simulink model "GaitAlgorithm_arduino_V1"  (R2024a)
settings: Solver=FixedStepAuto  StartTime=0.0  StopTime=inf  RelTol=1e-3  EnableMultiTasking=on
undefined symbols (not defined in the file): DiscIntNeverNeededParam
libraries: simulink x26, mcp2515lib x13, matrix_library x6, arduinolib x2, arduinosensorlib x2
(part 1 of 2)
settings Model: ExtModeTrigDuration=2  Creator=82108  LastModifiedBy=sejon
settings OptimizationCC: EnhancedBackFolding=on  PassReuseOutputArgsAs=Individual arguments  ZeroExternalMemoryAtStartup=off  ZeroInternalMemoryAtStartup=off  MaxStackSize=64  OptimizeBlockOrder=speed  DifferentSizesBufferReuse=on  OptimizationCustomize=off  EfficientTunableParamExpr=on
settings DebuggingCC: ParameterTunabilityLossMsg=error
settings HardwareCC: ProdBitPerInt=16  ProdBitPerPointer=16  ProdBitPerSizeT=16  ProdBitPerPtrDiffT=16  ProdLargestAtomicFloat=None  ProdWordSize=8  ProdHWDeviceType=Atmel->AVR  TargetBitPerPointer=64  TargetBitPerSizeT=64  TargetBitPerPtrDiffT=64  TargetLongLongMode=on  TargetIntDivRoundTo=Zero  TargetEndianess=LittleEndian  TargetWordSize=64  TargetHWDeviceType=Custom Processor->MATLAB Host Computer  ProdEqTarget=off
settings SFSimCC: MATLABDynamicMemAlloc=off
settings RTWCC: Description=Embedded Coder  SystemTargetFile=ert.tlc  HardwareBoard=Arduino Uno  TemplateMakefile=ert_default_tmf  Toolchain=Arduino AVR  BuildConfiguration=Faster Runs  GPUComputeCapability=3.5
settings CodeAppCC: ForceParamTrailComments=on  IgnoreCustomStorageClasses=off  OperatorAnnotations=on  SimulinkDataObjDesc=on  SFDataObjDesc=on  InsertBlockDesc=on
settings ERTTargetCC: SupportContinuousTime=on  SupportVariableSizeSignals=on  ExtModeTransport=3  ExtModeStaticAlloc=on  ExtModeAutomaticAllocSize=off  ExtModeStaticAllocSize=250  ExtModeMexFile=ext_xcp  ExtModeIntrfLevel=Level2 - Open

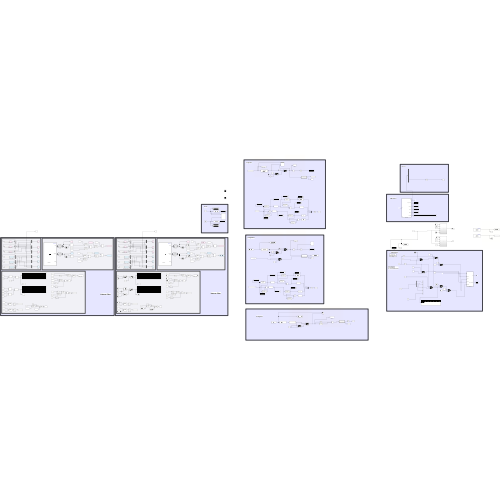
[thumbnail: Simulink's stored preview of the top-level diagram]
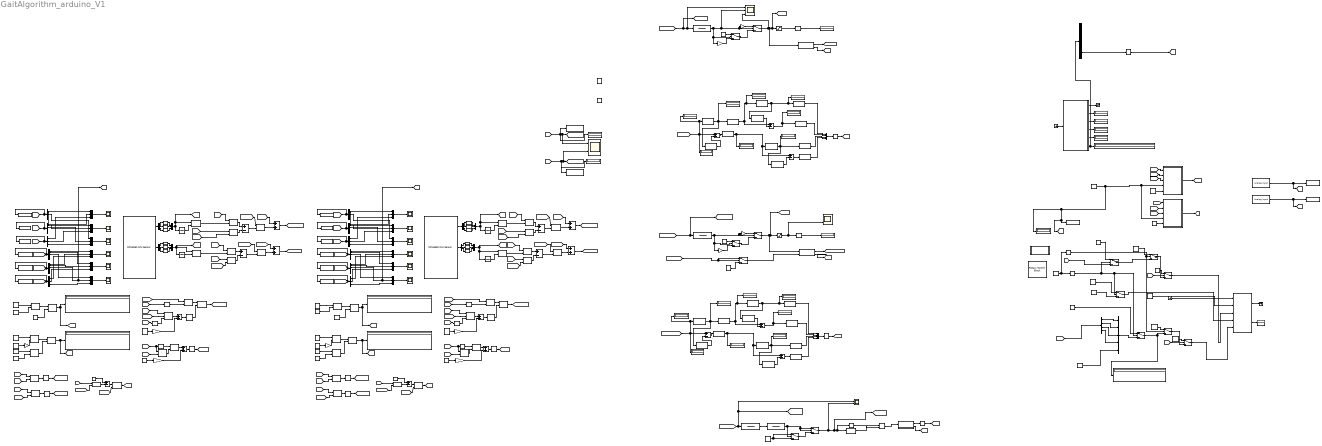
== system GaitAlgorithm_arduino_V1 ==
  note: D : Driving Mode
      | Z : Zeroing Mode
      | TZ : To zero Position Mode
  note: LIMIT STOP
  note: CAN Transmit
  note: DC Algorithm
  note: IC Algorithm
  note: Kalman Filter
  note: IMU data
  note: CAN Receive
  note: IC
  note: Kalman Filter
  note: LG Algorithm
  AND2 : Logic  IconShape=distinctive  AllPortsSameDT=off  OutDataTypeStr=boolean
  Acc_x : Scope
  Acc_x1 : Scope
  Acc_y : Scope
  Acc_y1 : Scope
  Acc_z : Scope
  Acc_z1 : Scope
  Add{,1,6,9..10,13..15} (8 alike) : Sum
  Add{2..5,7..8,11..12,16..19} (12 alike) : Sum  Inputs=+-
  Analog Input : arduinolib/Analog Input  pinNumber=0  ReadResultsOnly=off  ConversionTriggerSource=Software  ExternalTriggerType=uint32( 0 )  OutputDataType=uint16  EnableConversionCompleteNotify=off  EnableOuputStatus=off  SampleTime=0.01  blockPlatform=arduino
  Analog Input1 : arduinolib/Analog Input  pinNumber=1  ReadResultsOnly=off  ConversionTriggerSource=Software  ExternalTriggerType=uint32( 0 )  OutputDataType=uint16  EnableConversionCompleteNotify=off  EnableOuputStatus=off  SampleTime=0.01  blockPlatform=arduino
  Bias{,1..11} (12 alike) : Bias  SaturateOnIntegerOverflow=off
  CANbegin : Subsystem  TreatAsAtomicUnit=on  mask{TargetHardware=Arduino, Oscillator=8, CANSpeed=1000, CSpin=10}
      mask prompts: TargetHardware "Target Hardware"; Oscillator "Oscillator frequency(MHz)"; CANSpeed "CAN speed(kHz)"; CSpin "Chip Select Pin"
      mask init:
      | % Get this mask's handle
      | maskObj = Simulink.Mask.get(gcb);
      | 
      | % Get the selected value from mask parameter's option
      | str_TargetHard = char(maskObj.Parameters(1).TypeOptions(TargetHardware));
      | str_Osc = char(maskObj.Parameters(2).TypeOptions(Oscillator));
      | str_CANSpeed = char(maskObj.Parameters(3).TypeOptions(CANSpeed));
      | 
      | % Set Icon
      | str1 = sprintf('%s(Model)',str_TargetHard);
      | str2 = sprintf('Oscillator: %s(MHz)',str_Osc);
      | str3 = sprintf('CAN Bus Speed: %s(kHz)',str_CANSpeed);
      | str4 = sprintf('Chip Select pin: %d',CSpin);
      | 
      | % Set the values of Variant Subsystem
      | switch str_TargetHard
      |     case 'Arduino'
      |         str = [str1,'\n',str2,'\n',str3,'\n',str4];
      |         evalin('base',sprintf('CSpin = %d;',CSpin));        
      |         evalin('base','Hardware = 1;');
      |     case 'Raspberry Pi'
      |         str = [str1,'\n',str2,'\n',str3];
      |         evalin('base',sprintf('clear CSpin',CSpin));           
      |         evalin('base','Hardware = 2;');     
      | end  
      | 
      | % Get the CAN Configuration register's value from mask parameter's option
      | if str_Osc == '8' %[MHz]
      |     switch str_CANSpeed
      |         case '1000'
      |             BPR = 0; PHSEG1 = 0; PRSEG = 0; PHSEG2 = 0;
      |         case '500'
      |             BPR = 0; PHSEG1 = 2; PRSEG = 0; PHSEG2 = 2;
      |         case '250'
      |             BPR = 0; PHSEG1 = 6; PRSEG = 0; PHSEG2 = 6;
      |         case '125'
      |             BPR = 1; PHSEG1 = 6; PRSEG = 1; PHSEG2 = 5;
      |         case '100'
      |             BPR = 1; PHSEG1 = 7; PRSEG = 2; PHSEG2 = 7;
      |         case '83.3'
      |             BPR = 1; PHSEG1 = 7; PRSEG = 6; PHSEG2 = 7;
      |         case '62.5'
      |             BPR = 3; PHSEG1 = 6; PRSEG = 0; PHSEG2 = 6;
      |         case '50'
      |             BPR = 3; PHSEG1 = 7; PRSEG = 2; PHSEG2 = 7;
      |         case '33.3'
      |             BPR = 4; PHSEG1 = 7; PRSEG = 6; PHSEG2 = 7;
      |     end            
      | elseif str_Osc == '16' %[MHz]
      |     switch str_CANSpeed  
      |         case '1000'
      |             BPR = 0; PHSEG1 = 2; PRSEG = 0; PHSEG2 = 2;
      |         case '500'
      |             BPR = 0; PHSEG1 = 6; PRSEG = 0; PHSEG2 = 6;
      |         case '250'
      |             BPR = 1; PHSEG1 = 6; PRSEG = 1; PHSEG2 = 5;        
      |         case '125'
      |             BPR = 3; PHSEG1 = 6; PRSEG = 0; PHSEG2 = 6;
      |         case '100'
      |             BPR = 3; PHSEG1 = 7; PRSEG = 2; PHSEG2 = 7;
      |         case '83.3'
      |             BPR = 3; PHSEG1 = 7; PRSEG = 6; PHSEG2 = 7;
      |         case '62.5'
      |             BPR = 7; PHSEG1 = 6; PRSEG = 0; PHSEG2 = 6;
      |         case '50'
      |             BPR = 7; PHSEG1 = 7; PRSEG = 2; PHSEG2 = 7;
      |         case '33.3'
      |             BPR = 9; PHSEG1 = 7; PRSEG = 6; PHSEG2 = 7;        
      |     end   
      | end
      | % Set the CAN Configuration register's value
      | address2A = BPR;          % bit7-6 :SJW, bit5-0: BPR
      | address29 = 192 ...       % bit7: BTLMODE = 1, bit6:SAM = 1
      |             + 8*PHSEG1 ...% bit5-3: PHSEG1
      |             +PRSEG;       % bit2-0: PRSEG
      | address28 = 128 ...       % bit7: SOF = 1, bit6:WAKFIL = 0
      |             + PHSEG2;     % bit5-3: 0, bit2-0: PHSEG2
      settings: RTWSystemCode=Nonreusable function
      mask TypeOptions TargetHardware: Arduino | Raspberry Pi
      mask Callback TargetHardware:
      | if(strcmp(get_param(gcb,'TargetHardware'),'Arduino'))
      |     set_param(gcb,'MaskVisibilities',{'on','on','on','on'})
      | else
      |     set_param(gcb,'MaskVisibilities',{'on','on','on','off'})
      | end
      mask TypeOptions Oscillator: 8 | 16
      mask TypeOptions CANSpeed: 1000 | 500 | 250 | 125 | 100 | 83.3 | 62.5 | 50 | 33.3
      mask DialogControl DescGroupVar Prompt: Description
      mask DialogControl DescTextVar Prompt: This block must be executed only once when beginning CAN communication because MCP2515’s register needs to be configured. And the frequency of oscillator for MCP2515 is also needed because it effects to the setting parameters of MCP2515's register.
      mask Display: disp(str)
  CANreceive : Subsystem  TreatAsAtomicUnit=on
      mask DialogControl DescGroupVar Prompt: Description
      mask DialogControl DescTextVar Prompt: CANreceive outputs CAN data by converting MCP2515 RX buffer register’s values. In/Out ports are no use because they are used for controlling the execution order. CAN_Received outputs 1(CAN received) or -1( No message).
  CANtransmit : Subsystem  TreatAsAtomicUnit=on
      mask DialogControl DescGroupVar Prompt: Description
      mask DialogControl DescTextVar Prompt: CANtransmit inputs CAN data by converting MCP2515 TX buffer register’s values. In/Out ports are no use because they are used for controlling the execution order. CAN_Transmitted outputs 1(Success) or 2(Fail).
  Compare To Constant1 : simulink/Logic and Bit Operations/Compare To Constant  relop=>=  const=0  OutDataTypeStr=boolean
  Compare To Constant4 : simulink/Logic and Bit Operations/Compare To Constant  relop=>=  const=0  OutDataTypeStr=boolean
  Compare To Constant5 : simulink/Logic and Bit Operations/Compare To Constant  relop=>  const=-2  OutDataTypeStr=boolean
  Compare To Constant7 : simulink/Logic and Bit Operations/Compare To Constant  relop===  const=1  OutDataTypeStr=boolean
  Compare To Constant8 : simulink/Logic and Bit Operations/Compare To Constant  relop===  const=2  OutDataTypeStr=boolean
  Compare To Constant9 : simulink/Logic and Bit Operations/Compare To Constant  relop=>=  const=0xff  OutDataTypeStr=boolean
  Constant : Constant  Value=[0 0 0 0]  OutDataTypeStr=uint8
  Constant1 : Constant  OutDataTypeStr=uint8
  Constant10 : Constant  Value=[0 0 0; 0 0 0; 0 0 0]  SampleTime=-1
  Constant11 : Constant  Value=[0 0 0; 0 0 0; 0 0 0]
  Constant12 : Constant  Value=[0 0 0 0 0 0; 0 0 0 0 0 0; 0 0 0 0 0 0]
  Constant13 : Constant  Value=[0 0 0; 0 0 0; 0 0 0]
  Constant14 : Constant  Value=0x168  OutDataTypeStr=uint16
  Constant15 : Constant  Value=[0x00 0x00 0x07 0xd0 ]  OutDataTypeStr=uint16
  Constant16 : Constant  Value=-1
  Constant17 : Constant  Value=-1
  Constant18 : Constant  Value=-2
  Constant19 : Constant  Value=3  SampleTime=0.01
  Constant21 : Constant  Value=0x468
  Constant22 : Constant  Value=[0 0 0 0 0 0 0 0 ]  OutDataTypeStr=uint8
  Constant23 : Constant  Value=0x468
  Constant24 : Constant  Value=[0 0 0 0 0 0 0 0 ]  OutDataTypeStr=uint8
  Constant25 : Constant  Value=2
  Constant3 : Constant  Value=4  OutDataTypeStr=uint8
  Constant4 : Constant  Value=-10
  Constant5 : Constant  Value=0x568
  Constant6 : Constant  OutDataTypeStr=uint8
  Constant7 : Constant  Value=[0x01 0 0 0 0 0 0 0]  OutDataTypeStr=uint8
  Constant8 : Constant  Value=[0 0 0; 0 0 0; 0 0 0]
  Constant9 : Constant  Value=[0 0 0 0 0 0; 0 0 0 0 0 0; 0 0 0 0 0 0]  SampleTime=-1
  Data Store Memory : DataStoreMemory  DataStoreName=T_G_Z  WriteAfterWriteMsg=warning  ShowAdditionalParam=off
  Data Store Memory1 : DataStoreMemory  DataStoreName=S_G_Z  WriteAfterWriteMsg=warning  ShowAdditionalParam=off
  Data Store Write : DataStoreWrite  DataStoreName=T_G_Z  DataStoreElements=T_G_Z  IndexOptions=Index vector (dialog)  Indices=1  OutputSizes=1
  Data Store Write1 : DataStoreWrite  DataStoreName=S_G_Z  DataStoreElements=S_G_Z  IndexOptions=Index vector (dialog)  Indices=1  OutputSizes=1
  Data Type Conversion{1..2,10..11} (4 alike) : DataTypeConversion  OutDataTypeStr=uint16  SaturateOnIntegerOverflow=off  RndMeth=Floor
  Data Type Conversion{6..7,9,12} (4 alike) : DataTypeConversion  OutDataTypeStr=uint8  SaturateOnIntegerOverflow=off  RndMeth=Floor
  Data Type Conversion{3..5,8} (4 alike) : DataTypeConversion  OutDataTypeStr=uint8  RndMeth=Floor
  Delay1 : Delay  DelayLength=1
  Delay2 : Delay  DelayLength=1
  Delay_acc : Delay  DelayLength=1  InitialCondition=[0; 0; 0; 0; 0;0]
  Delay_acc1 : Delay  DelayLength=1  InitialCondition=[0; 0; 0; 0; 0;0]
  Delay_gyro : Delay  DelayLength=1  InitialCondition=[0; 0; 0; 0; 0;0]
  Delay_gyro1 : Delay  DelayLength=1  InitialCondition=[0; 0; 0; 0; 0;0]
  Demux : Demux  Outputs=8
  Demux{3..4,6..7,9..10,16,18} (8 alike) : Demux  Outputs=6
  Demux{5,8,11..15,17} (8 alike) : Demux  Outputs=3
  Demux2 : Demux
  Detect Increase1 : simulink/Logic and Bit Operations/Detect Increase  vinit=0.0  OutDataTypeStr=boolean
  Discrete-Time Integrator{,1..3} (4 alike) : DiscreteIntegrator  SampleTime=-1  ICPrevOutput=DiscIntNeverNeededParam  ICPrevScaledInput=DiscIntNeverNeededParam
  Display{1..24,27..33} (31 alike) : Display
      Display11 settings: Format=hex (Stored Integer)
      Display12 settings: Format=hex (Stored Integer)
      Display13 settings: Format=hex (Stored Integer)
      Display14 settings: Format=hex (Stored Integer)
      Display15 settings: Format=hex (Stored Integer)
      Display16 settings: Format=hex (Stored Integer)
      Display17 settings: Format=hex (Stored Integer)
      Display18 settings: Format=hex (Stored Integer)
      Display19 settings: Format=hex (Stored Integer)
      Display20 settings: Format=hex (Stored Integer)
      Display21 settings: Format=hex (Stored Integer)
      Display22 settings: Format=hex (Stored Integer)
      Display23 settings: Format=hex (Stored Integer)
      Display24 settings: Format=hex (Stored Integer)
      Display28 settings: Format=hex (Stored Integer)
      Display30 settings: Format=hex (Stored Integer)
      Display32 settings: Format=hex (Stored Integer)
      Display7 settings: Format=hex (Stored Integer)
      Display9 settings: Format=hex (Stored Integer)
  Enabled Subsystem1 : Subsystem  TreatAsAtomicUnit=on
  Enabled Subsystem3 : Subsystem  TreatAsAtomicUnit=on
  Enabled Subsystem4 : Subsystem  TreatAsAtomicUnit=on
  Gain : Gain  Gain=-0.01
  Gain1 : Gain  Gain=-0.01
  Gain{2..5} (4 alike) : Gain  Gain=2
  Ground : Ground
  Ground1 : Ground
  Gyro_x : Scope
  Gyro_x1 : Scope
  Gyro_y : Scope
  Gyro_y1 : Scope
  Gyro_z : Scope
  Gyro_z1 : Scope
  IdentityMatrix{,1..2,4,7..9,11} (8 alike) : IdentityMatrix  OutputDimensions=3  SampleTime=-1
  IdentityMatrix{3,5..6,10,12..13} (6 alike) : IdentityMatrix  OutputDimensions=6  SampleTime=-1
  MPU6050 IMU Sensor : arduinosensorlib/MPU6050 IMU Sensor  I2CModule=0  SlaveAddress=0x68  Accel=on  AngularRate=on  Temperature=off  Status=on  Timestamp=off  EulerAngles=off  Quat=off  AccelRange=2G  GyroRange=250 dps  DmpOdr=200 Hz  Dlpf=Accelerometer: 184Hz, Gyroscope: 188Hz  spf=1  SampleTime=0.01  QueueSizeFactor=1
  MPU6050 IMU Sensor1 : arduinosensorlib/MPU6050 IMU Sensor  I2CModule=0  SlaveAddress=0x69  Accel=on  AngularRate=on  Temperature=off  Status=on  Timestamp=off  EulerAngles=off  Quat=off  AccelRange=2G  GyroRange=250 dps  DmpOdr=200 Hz  Dlpf=Accelerometer: 184Hz, Gyroscope: 188Hz  spf=1  SampleTime=0.01  QueueSizeFactor=1
  Matrix Concatenate{,1,4,7..8,11} (6 alike) : Concatenate  Mode=Multidimensional array  ConcatenateDimension=2
  Matrix Concatenate{2..3,5..6,9..10,12..13} (8 alike) : Concatenate  Mode=Multidimensional array
  Matrix Divide : Product  Inputs=/  Multiplication=Matrix(*)
  Matrix Divide1 : Product  Inputs=/  Multiplication=Matrix(*)
  Matrix Multiply{,1..3,5..23,25..29} (28 alike) : Product  Multiplication=Matrix(*)
  Matrix Multiply24 : Product  Inputs=3  Multiplication=Matrix(*)
  Matrix Multiply4 : Product  Inputs=3  Multiplication=Matrix(*)
  Mux{,1..15} (16 alike) : Mux  Inputs=3
  Reshape1 : Reshape
  Reshape2 : Reshape
  Reshape3 : Reshape
  Rotary Switch : RotarySwitchBlock
      settings: Values={{'D', 'Z', 'TZ'}, [0 1 2]}
  Saturation1 : Saturate  UpperLimit=200  LowerLimit=-100
  Saturation3 : Saturate  UpperLimit=200  LowerLimit=-100
  Scope : Scope  NumInputPorts=2
  Scope1 : Scope  NumInputPorts=2
  Scope3 : Scope  NumInputPorts=3
  Scope4 : Scope  NumInputPorts=2
  Shift Arithmetic{1,7,10..11} (4 alike) : ArithShift  BitShiftNumber=8  BitShiftDirection=Right
  Shift Arithmetic13 : ArithShift  BitShiftNumber=16  BitShiftDirection=Right
  Shift Arithmetic{2,4,6,9} (4 alike) : ArithShift  BitShiftNumber=8  BitShiftDirection=Left
  Shift Arithmetic3 : ArithShift  BitShiftNumber=16  BitShiftDirection=Left
  Shift Arithmetic5 : ArithShift  BitShiftNumber=16  BitShiftDirection=Right
  Shift Arithmetic8 : ArithShift  BitShiftNumber=16  BitShiftDirection=Left
  Subsystem : Subsystem
  Subsystem1 : Subsystem
  Switch{,1..4,11..12} (7 alike) : Switch  Criteria=u2 > Threshold  SaturateOnIntegerOverflow=off  InputSameDT=off
  Switch10 : Switch  Threshold=2  SaturateOnIntegerOverflow=off  InputSameDT=off
  Switch13 : Switch  Criteria=u2 > Threshold  Threshold=25  SaturateOnIntegerOverflow=off  InputSameDT=off
  Switch5 : Switch  Criteria=u2 > Threshold  Threshold=40  SaturateOnIntegerOverflow=off  InputSameDT=off
  Switch6 : Switch  Criteria=u2 > Threshold  Threshold=-40  SaturateOnIntegerOverflow=off  InputSameDT=off
  Switch7 : Switch  Criteria=u2 > Threshold  Threshold=10  SaturateOnIntegerOverflow=off  InputSameDT=off
  Switch8 : Switch  Criteria=u2 > Threshold  Threshold=-10  SaturateOnIntegerOverflow=off  InputSameDT=off
  Switch9 : Switch  Threshold=-2  SaturateOnIntegerOverflow=off  InputSameDT=off
  Terminator : Terminator
  Terminator1 : Terminator
  To Workspace : ToWorkspace  VariableName=predicted_acc  SaveFormat=Timeseries  SampleTime=-1
  To Workspace1 : ToWorkspace  VariableName=measured_acc  SaveFormat=Timeseries  SampleTime=-1
  To Workspace10 : ToWorkspace  VariableName=estimated_gyro_shank  SaveFormat=Timeseries  SampleTime=-1
  To Workspace11 : ToWorkspace  VariableName=measured_gyro_shank  SaveFormat=Timeseries  SampleTime=-1
  To Workspace12 : ToWorkspace  VariableName=UDPsig  SaveFormat=Timeseries  SampleTime=-1
  To Workspace13 : ToWorkspace  VariableName=emg0  SaveFormat=Timeseries  SampleTime=-1
  To Workspace14 : ToWorkspace  VariableName=emg1  SaveFormat=Timeseries  SampleTime=-1
  To Workspace2 : ToWorkspace  VariableName=estimated_acc  SaveFormat=Timeseries  SampleTime=-1
  To Workspace3 : ToWorkspace  VariableName=predicted_gyro  SaveFormat=Timeseries  SampleTime=-1
  To Workspace4 : ToWorkspace  VariableName=estimated_gyro  SaveFormat=Timeseries  SampleTime=-1
  To Workspace5 : ToWorkspace  VariableName=measured_gyro  SaveFormat=Timeseries  SampleTime=-1
  To Workspace6 : ToWorkspace  VariableName=predicted_acc_shank  SaveFormat=Timeseries  SampleTime=-1
  To Workspace7 : ToWorkspace  VariableName=measured_acc_shank  SaveFormat=Timeseries  SampleTime=-1
  To Workspace8 : ToWorkspace  VariableName=estimated_acc_shank  SaveFormat=Timeseries  SampleTime=-1
  To Workspace9 : ToWorkspace  VariableName=predicted_gyro_shank  SaveFormat=Timeseries  SampleTime=-1
  Transfer Fcn1 : TransferFcn  Denominator=[0.029 1]
  Transfer Fcn18 : TransferFcn  Numerator=[0.018 0]  Denominator=[0.018 1]
  Transfer Fcn19 : TransferFcn  Denominator=[0.08 1]
  Transfer Fcn2 : TransferFcn  Denominator=[0.029 1]
  Transpose{,1..5} (6 alike) : matrix_library/Transpose
  UDP : Display
  Vector Concatenate1 : Concatenate  NumInputs=4  ConcatenateDimension=2
  Vector Concatenate2 : Concatenate  NumInputs=4  ConcatenateDimension=2
  Vector Concatenate3 : Concatenate  NumInputs=5
  sensor noise : Gain  Gain=0.03
  sensor noise1 : Gain  Gain=0.03
  system noise : Gain  Gain=0.005
  system noise1 : Gain  Gain=0.005
  wires:
  Data Type Conversion10/1 -> Add2/1, Display21/1, Shift Arithmetic11/1
  Data Type Conversion7/1 -> Vector Concatenate2/1
  Add3/1 -> Data Type Conversion11/1
  Vector Concatenate2/1 -> Reshape2/1
  Shift Arithmetic4/1 -> Add4/2
  Shift Arithmetic13/1 -> Shift Arithmetic3/1, Display7/1, Data Type Conversion10/1
  [to_shift_IC] -> Add3/1, Display28/1, Display20/1, Shift Arithmetic13/1
  Shift Arithmetic11/1 -> Shift Arithmetic2/1, Display18/1, Data Type Conversion7/1
  Shift Arithmetic2/1 -> Add2/2
  Data Type Conversion6/1 -> Vector Concatenate2/4
  Shift Arithmetic7/1 -> Shift Arithmetic4/1, Display23/1, Data Type Conversion5/1
  Data Type Conversion5/1 -> Vector Concatenate2/3
  Shift Arithmetic3/1 -> Add3/2
  Data Type Conversion11/1 -> Display19/1, Add4/1, Shift Arithmetic7/1
  Add2/1 -> Data Type Conversion4/1, Display22/1
  Data Type Conversion4/1 -> Vector Concatenate2/2
  Add4/1 -> Data Type Conversion6/1
  [TGZ] -> Data Store Write/1, Display3/1, Scope1/2, [thigh_gyro_z]
  [SGZ] -> Display2/1, Scope1/1, [shank_gyro_z], Data Store Write1/1
  Demux2/4 -> Vector Concatenate3/4
  [pos] -> Demux2/1
  Demux2/1 -> Vector Concatenate3/1
  Demux2/3 -> Vector Concatenate3/3
  Demux2/2 -> Vector Concatenate3/2
  Constant/1 -> Vector Concatenate3/5
  CANtransmit/1(Out) -> Terminator/1
  Constant1/1 -> CANtransmit/2(CAN_ext)
  CANtransmit/2(CAN_Transmitted) -> Display1/1
  Switch/1 -> Switch3/3
  Constant5/1 -> Switch/1
  Constant3/1 -> Switch1/3
  Switch1/1 -> CANtransmit/4(CAN_dlc)
  Constant6/1 -> Switch1/1
  Vector Concatenate3/1 -> Switch2/3
  Constant7/1 -> Switch2/1
  Switch2/1 -> Display9/1, Switch4/3
  Compare To Constant7/1 -> Switch/2, Switch2/2, Switch1/2
  Add16/1 -> Matrix Multiply28/2
  Mux3/1 -> Gyro_x/1
  [AR_x_bar] -> Add9/1
  [AR_x_bar] -> Matrix Multiply12/2
  Demux6/2 -> Mux4/1
  Demux8/2 -> Mux4/3
  Demux7/3 -> [SGZ], Mux5/2
  [AR_x] -> To Workspace5/1, Demux8/1
  Matrix Multiply13/1 -> Add9/2
  Transpose3/1 -> Matrix Multiply22/1
  [kalmangain] -> Matrix Multiply13/1
  Demux5/3 -> Mux2/3
  [x_hat] -> To Workspace2/1, Demux4/1
  Demux3/3 -> Mux2/1
  Matrix Multiply11/1 -> Add8/1
  Demux5/2 -> Mux1/3
  Matrix Multiply9/1 -> Add7/2
  Add1/1 -> Matrix Divide/1
  Transpose2/1 -> Matrix Multiply4/3
  Matrix Multiply3/1 -> Matrix Multiply5/1
  [H] -> Transpose1/1
  [H] -> Matrix Multiply/1
  [H] -> Matrix Multiply7/1
  [x_hat] -> Matrix Multiply6/2
  Transpose1/1 -> Matrix Multiply3/2
  Matrix Divide/1 -> Matrix Multiply5/2
  [cov_bar] -> Matrix Multiply3/1
  Delay_acc/1 -> [x_bar]
  Matrix Multiply5/1 -> [kalmangain]
  Matrix Concatenate1/1 -> Matrix Concatenate2/2
  [H] -> Transpose2/1
  IdentityMatrix3/1 -> system noise/1
  Gain/1 -> Matrix Concatenate/2
  Matrix Concatenate4/1 -> Matrix Concatenate6/1
  [cov] -> Matrix Multiply1/2
  Constant10/1 -> Matrix Concatenate4/2
  Delay1/1 -> [cov_bar]
  Matrix Concatenate3/1 -> Matrix Multiply/2
  [C_Phi] -> Matrix Multiply1/1, Transpose/1
  [x_bar] -> Demux3/1, To Workspace/1
  Matrix Concatenate2/1 -> [C_Phi], Display5/1
  [AR_x_bar] -> To Workspace3/1, Demux6/1
  Matrix Concatenate6/1 -> [H], Display4/1
  Mux7/1 -> Acc_y1/1
  system noise/1 -> Add/2
  Demux8/3 -> Mux5/3
  system noise1/1 -> Add14/2
  [C_Phi] -> Matrix Multiply14/1
  Mux/1 -> Acc_x/1
  [H_2] -> Matrix Multiply18/1
  Constant9/1 -> Matrix Concatenate6/2
  Mux2/1 -> Acc_z/1
  Demux11/1 -> Mux9/3
  Matrix Multiply4/1 -> Add1/1
  [x_hat_2] -> To Workspace8/1, Demux16/1
  Demux4/2 -> Mux1/2
  Bias7/1 -> Mux14/1
  [H] -> Matrix Multiply11/1
  [H_2] -> Transpose4/1
  Matrix Concatenate10/1 -> Matrix Multiply15/2
  IdentityMatrix2/1 -> Matrix Concatenate1/2
  Matrix Multiply26/1 -> Delay_acc1/1
  [cov_bar_2] -> Matrix Multiply24/2
  Mux4/1 -> Gyro_y/1
  MPU6050 IMU Sensor1/1 -> Demux13/1  "x_now"
  [cov_bar_2] -> Matrix Multiply23/1
  sensor noise/1 -> Add1/2
  Mux15/1 -> Matrix Concatenate12/1, Discrete-Time Integrator3/1, [AR_x_2]
  Matrix Multiply8/1 -> Add6/2
  Matrix Multiply15/1 -> Add16/1
  Discrete-Time Integrator1/1 -> Matrix Concatenate5/2
  Demux9/2 -> Mux7/1
  [x_bar] -> Matrix Multiply7/2
  Mux8/1 -> Acc_z1/1
  [C_Phi] -> Matrix Multiply6/1
  Demux10/1 -> Mux9/2
  [x_bar_2] -> Demux9/1, To Workspace6/1
  Demux6/1 -> Mux3/1
  IdentityMatrix1/1 -> Gain/1
  Matrix Multiply22/1 -> Add14/1
  [AR_x_hat] -> To Workspace4/1, Demux7/1
  Bias9/1 -> Mux15/2
  Demux4/1 -> Mux/2
  Transpose4/1 -> Matrix Multiply23/2
  Bias10/1 -> Mux15/1
  Demux15/2 -> Bias9/1
  Demux8/1 -> Mux3/3
  Mux6/1 -> Acc_x1/1
  Bias11/1 -> Mux15/3
  Add13/1 -> [AR_x_hat_2]
  Demux6/3 -> Mux5/1
  Delay2/1 -> [cov_bar_2]
  Demux18/2 -> Mux10/1
  Bias8/1 -> Mux14/3
  Matrix Multiply24/1 -> Add15/1
  [AR_x_hat] -> Matrix Multiply14/2
  Mux13/1 -> [x_2], Matrix Concatenate10/1, Discrete-Time Integrator2/1
  IdentityMatrix11/1 -> Matrix Concatenate11/1
  [cov_bar] -> Matrix Multiply4/2
  Demux15/1 -> Bias10/1
  IdentityMatrix9/1 -> Matrix Concatenate8/2
  Demux14/1 -> Bias7/1
  Matrix Multiply20/1 -> Add13/2
  Mux1/1 -> Acc_y/1
  Demux3/2 -> Mux1/1
  Demux13/2 -> Bias3/1
  Bias6/1 -> Mux14/2
  Demux14/2 -> Bias6/1
  IdentityMatrix/1 -> Matrix Concatenate/1
  Demux4/3 -> Mux2/2
  Matrix Multiply6/1 -> Delay_acc/1
  [kalmangain] -> Matrix Multiply9/2
  Bias5/1 -> Mux13/3
  Bias3/1 -> Mux13/2
  Add5/1 -> Matrix Multiply8/2
  Bias2/1 -> Mux12/3
  Add7/1 -> Matrix Multiply10/1
  Constant8/1 -> Matrix Concatenate1/1
  Demux12/3 -> Bias2/1
  Demux12/1 -> Bias1/1
  Demux13/3 -> Bias5/1
  Add12/1 -> Matrix Multiply20/2
  [AR_x_hat_2] -> Matrix Multiply21/2
  Bias4/1 -> Mux13/1
  IdentityMatrix6/1 -> Add7/1
  Discrete-Time Integrator2/1 -> Matrix Concatenate10/2
  Bias1/1 -> Mux12/1
  [kalmangain] -> Matrix Multiply8/1
  MPU6050 IMU Sensor/1 -> Demux12/1  "x_now"
  Add8/1 -> Matrix Multiply13/2
  [kalmangain_2] -> Matrix Multiply20/1
  Add6/1 -> [x_hat]
  Matrix Multiply2/1 -> Add/1
  Demux14/3 -> Bias8/1
  Matrix Divide1/1 -> Matrix Multiply25/2
  Demux9/3 -> Mux8/1
  Matrix Multiply16/1 -> Matrix Multiply22/2
  [AR_x_2] -> To Workspace11/1, Demux11/1
  Demux17/1 -> Mux6/3
  [x_2] -> To Workspace7/1, Demux17/1
  Mux14/1 -> Matrix Concatenate5/1, [AR_x], Discrete-Time Integrator1/1
  Demux9/1 -> Mux6/1
  Matrix Concatenate11/1 -> Matrix Concatenate13/1
  sensor noise1/1 -> Add15/2
  Demux7/2 -> Mux4/2
  Demux12/2 -> Bias/1
  Matrix Multiply19/1 -> Add12/2
  [x_bar] -> Add6/1
  Matrix Multiply27/1 -> Add16/2
  [cov_2] -> Matrix Multiply16/2
  Matrix Multiply12/1 -> Add8/2
  Bias/1 -> Mux12/2
  Matrix Multiply18/1 -> Add12/1
  Matrix Multiply21/1 -> Delay_gyro1/1
  [H_2] -> Matrix Multiply29/1
  Delay_gyro1/1 -> [AR_x_bar_2]
  Demux16/3 -> Mux8/2
  Add14/1 -> Delay2/1
  Transpose5/1 -> Matrix Multiply24/3
  [H_2] -> Matrix Multiply27/1
  Demux15/3 -> Bias11/1
  [x_hat_2] -> Matrix Multiply26/2
  Matrix Multiply25/1 -> [kalmangain_2]
  Matrix Multiply23/1 -> Matrix Multiply25/1
  [cov_bar_2] -> Matrix Multiply17/2
  [H] -> Matrix Multiply12/1
  [C_Phi_2] -> Matrix Multiply26/1
  [C_Phi_2] -> Matrix Multiply16/1, Transpose3/1
  IdentityMatrix13/1 -> Add11/1
  [H_2] -> Matrix Multiply19/1
  Constant11/1 -> Matrix Concatenate8/1
  MPU6050 IMU Sensor1/2 -> Demux15/1  "x_now_AR"
  Add/1 -> Delay1/1
  Delay_gyro/1 -> [AR_x_bar]
  Demux18/1 -> Mux9/1
  Mux11/1 -> Gyro_z1/1
  Discrete-Time Integrator3/1 -> Matrix Concatenate12/2
  Demux13/1 -> Bias4/1
  [AR_x_bar_2] -> Matrix Multiply19/2
  [AR_x_bar_2] -> To Workspace9/1, Demux18/1
  [AR_x_hat_2] -> To Workspace10/1, Demux10/1
  IdentityMatrix12/1 -> sensor noise1/1
  Mux12/1 -> [x], Matrix Concatenate3/1, Discrete-Time Integrator/1
  Discrete-Time Integrator/1 -> Matrix Concatenate3/2
  Demux10/2 -> Mux10/2
  [AR_x_bar_2] -> Add13/1
  Demux18/3 -> Mux11/1
  Matrix Concatenate13/1 -> [H_2], Display6/1
  Matrix Concatenate/1 -> Matrix Concatenate2/1
  Demux7/1 -> Mux3/2
  Mux10/1 -> Gyro_y1/1
  [kalmangain_2] -> Matrix Multiply29/2
  IdentityMatrix4/1 -> Matrix Concatenate4/1
  [x_bar_2] -> Add10/1
  IdentityMatrix10/1 -> system noise1/1
  [H] -> Matrix Multiply9/1
  Mux5/1 -> Gyro_z/1
  IdentityMatrix7/1 -> Matrix Concatenate7/1
  Matrix Concatenate5/1 -> Matrix Multiply11/2
  Matrix Concatenate7/1 -> Matrix Concatenate9/1
  Matrix Multiply1/1 -> Matrix Multiply2/2
  Demux10/3 -> [TGZ], Mux11/2
  Matrix Multiply14/1 -> Delay_gyro/1
  Gain1/1 -> Matrix Concatenate7/2
  Demux3/1 -> Mux/1
  Matrix Concatenate12/1 -> Matrix Multiply18/2
  [H] -> Matrix Multiply4/1
  Matrix Concatenate8/1 -> Matrix Concatenate9/2
  Delay_acc1/1 -> [x_bar_2]
  Mux9/1 -> Gyro_x1/1
  [kalmangain_2] -> Matrix Multiply28/1
  Add11/1 -> Matrix Multiply17/1
  IdentityMatrix5/1 -> sensor noise/1
  Add9/1 -> [AR_x_hat]
  Demux17/2 -> Mux7/3
  [cov_bar] -> Matrix Multiply10/2
  [C_Phi_2] -> Matrix Multiply21/1
  Add15/1 -> Matrix Divide1/1
  Add10/1 -> [x_hat_2]
  Demux17/3 -> Mux8/3
  Demux11/3 -> Mux11/3
  [x] -> To Workspace1/1, Demux5/1
  [H_2] -> Matrix Multiply24/1
  Constant13/1 -> Matrix Concatenate11/2
  IdentityMatrix8/1 -> Gain1/1
  Matrix Multiply29/1 -> Add11/2
  [x_bar_2] -> Matrix Multiply27/2
  Matrix Multiply7/1 -> Add5/2
  Matrix Multiply/1 -> Add5/1
  [H_2] -> Transpose5/1
  Demux16/1 -> Mux6/2
  Matrix Multiply17/1 -> [cov_2]
  Constant12/1 -> Matrix Concatenate13/2
  Demux11/2 -> Mux10/3
  Demux16/2 -> Mux7/2
  Demux5/1 -> Mux/3
  MPU6050 IMU Sensor/2 -> Demux14/1  "x_now_AR"
  Matrix Concatenate9/1 -> [C_Phi_2], Display8/1
  Matrix Multiply10/1 -> [cov]
  [H_2] -> Matrix Multiply15/1
  Transpose/1 -> Matrix Multiply2/1
  Matrix Multiply28/1 -> Add10/2
  Ground/1 -> CANtransmit/1(In)
  Reshape2/1 -> [pos_IC]
  CANreceive/1(Out) -> Terminator1/1
  Ground1/1 -> CANreceive/1(In)
  CANreceive/2(CAN_Received) -> Display27/1
  CANreceive/3(CAN_ext) -> Display29/1
  CANreceive/4(CAN_id) -> Display30/1
  CANreceive/5(CAN_dlc) -> Display31/1
  CANreceive/6(CAN_data) -> Demux/1, Display32/1
  Gain5/1 -> Switch8/3
  [shank_gyro_z] -> [IC_IMU_PreF], Transfer Fcn2/1
  Constant17/1 -> Switch8/1
  Gain4/1 -> Switch7/1
  Switch8/1 -> Switch7/3
  Transfer Fcn2/1 -> Switch8/2, Gain5/1, Gain4/1, Switch7/2
  Switch7/1 -> Enabled Subsystem4/1(In1), [IC_IMU], Saturation3/1
  Compare To Constant4/1 -> Display33/1
  Saturation3/1 -> Compare To Constant4/1, Scope4/2
  Enabled Subsystem4/2(Out2) -> [id_ic]
  Enabled Subsystem4/1(Out1) -> [to_shift_IC]
  [shank_gyro_z] -> [DC_IMU_PreF], Scope/1, Transfer Fcn18/1
  Transfer Fcn18/1 -> Transfer Fcn19/1
  Transfer Fcn19/1 -> Switch9/2, Switch10/2, Switch10/1
  Switch10/1 -> Scope/2, [DC_IMU], Compare To Constant5/1, Detect Increase1/1
  Compare To Constant5/1 -> AND2/1
  Detect Increase1/1 -> AND2/2
  AND2/1 -> Enabled Subsystem3/1(In2)
  Enabled Subsystem3/1(Out1) -> Reshape3/1
  Enabled Subsystem3/2(Out2) -> [id_dc]
  [pos_DC] -> Subsystem/1(In1)
  [id_dc] -> Subsystem1/1(In1)
  [pos_IC] -> Subsystem/2(In2)
  [id_ic] -> Subsystem1/2(In2)
  [pos_lg] -> Subsystem/3(In3)
  Constant15/1 -> Subsystem/5(In6)
  Constant14/1 -> Subsystem1/5(In6)
  Subsystem/1(Out1) -> [pos]
  Subsystem1/1(Out1) -> [id]
  [id_lg] -> Subsystem1/3(In3)
  Reshape3/1 -> [pos_DC]
  Compare To Constant8/1 -> Switch4/2, Switch3/2
  Constant21/1 -> Switch3/1
  Constant22/1 -> Switch4/1
  Switch9/1 -> Switch10/3
  Constant18/1 -> Switch9/1, Switch9/3
  [id] -> Switch/3
  [LS_ID] -> Switch12/2
  Switch4/1 -> Switch12/3
  Constant24/1 -> Switch12/1
  [LS_ID] -> Switch11/2
  Constant23/1 -> Switch11/1
  Switch3/1 -> Switch11/3
  Constant25/1 -> Compare To Constant8/1, Compare To Constant7/1
  [thigh_gyro_z] -> Switch13/1, Switch13/2
  Constant4/1 -> Switch13/3
  Switch13/1 -> Enabled Subsystem4/2(In2)
  Gain3/1 -> Switch6/3
  Reshape1/1 -> [pos_lg]
  Data Type Conversion2/1 -> Display12/1, Add19/1, Shift Arithmetic10/1
  Shift Arithmetic1/1 -> Shift Arithmetic6/1, Display11/1, Data Type Conversion12/1
  Compare To Constant1/1 -> Display10/1
  Vector Concatenate1/1 -> Reshape1/1
  Shift Arithmetic9/1 -> Add19/2
  Enabled Subsystem1/2(Out2) -> [id_lg]
  Constant16/1 -> Switch6/1
  Switch6/1 -> Switch5/3
  Saturation1/1 -> Compare To Constant1/1
  Add19/1 -> Data Type Conversion9/1
  [shank_gyro_z] -> [LG_IMU_PreF], Scope3/1, Transfer Fcn1/1
  Data Type Conversion12/1 -> Vector Concatenate1/1
  Shift Arithmetic5/1 -> Shift Arithmetic8/1, Display24/1, Data Type Conversion1/1
  [to_shift_lg] -> Add18/1, Display17/1, Display13/1, Shift Arithmetic5/1
  Add18/1 -> Data Type Conversion2/1
  Gain2/1 -> Switch5/1
  Data Type Conversion8/1 -> Vector Concatenate1/3
  Data Type Conversion1/1 -> Add17/1, Display14/1, Shift Arithmetic1/1
  Data Type Conversion9/1 -> Vector Concatenate1/4
  Transfer Fcn1/1 -> Switch6/2, Gain3/1, Scope3/2, Gain2/1, Switch5/2
  Shift Arithmetic8/1 -> Add18/2
  Data Type Conversion3/1 -> Vector Concatenate1/2
  Shift Arithmetic10/1 -> Shift Arithmetic9/1, Display16/1, Data Type Conversion8/1
  Switch5/1 -> Scope3/3, Enabled Subsystem1/1(In1), [LG_IMU], Saturation1/1
  Enabled Subsystem1/1(Out1) -> [to_shift_lg]
  Add17/1 -> Data Type Conversion3/1, Display15/1
  Shift Arithmetic6/1 -> Add17/2
  Demux/7 -> Compare To Constant9/1
  Compare To Constant9/1 -> [LS_ID]
  Switch11/1 -> CANtransmit/3(CAN_id)
  Switch12/1 -> CANtransmit/5(CAN_data)
  Analog Input/1 -> [emg0], To Workspace13/1
  Analog Input1/1 -> [emg1], To Workspace14/1
  Constant19/1 -> [UDPsig], To Workspace12/1, UDP/1, Subsystem1/4(In5), Subsystem/4(In5)

== system GaitAlgorithm_arduino_V1/CANbegin ==
  Constant : Constant  Value=0  OutDataTypeStr=boolean  SampleTime=-1
  Temporary buffer : DataStoreMemory  DataStoreName=temp_1byte  ReadBeforeWriteMsg=warning  WriteAfterWriteMsg=warning  WriteAfterReadMsg=warning  ShowAdditionalParam=off  OutDataTypeStr=uint8
  Unit Delay : UnitDelay  InitialCondition=1  SampleTime=-1  HasFrameUpgradeWarning=on
  setup : Subsystem  TreatAsAtomicUnit=on
      settings: RTWSystemCode=Nonreusable function  RTWFileNameOpts=Use subsystem name
  wires:
  Unit Delay/1 -> setup/Enable
  Constant/1 -> Unit Delay/1

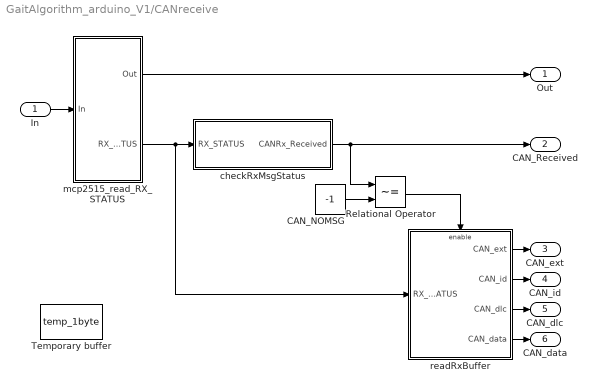
== system GaitAlgorithm_arduino_V1/CANreceive ==
  In : Inport
  CAN_NOMSG : Constant  Value=-1  OutDataTypeStr=int8
  Relational Operator : RelationalOperator  Operator=~=  OutDataTypeStr=boolean  InputSameDT=off
  Temporary buffer : DataStoreMemory  DataStoreName=temp_1byte  ReadBeforeWriteMsg=warning  WriteAfterWriteMsg=warning  WriteAfterReadMsg=warning  ShowAdditionalParam=off  OutDataTypeStr=uint8
  checkRxMsgStatus : Subsystem  TreatAsAtomicUnit=on
  mcp2515_read_RX_STATUS : Subsystem  TreatAsAtomicUnit=on
  readRxBuffer : Subsystem  TreatAsAtomicUnit=on
  Out : Outport
  CAN_Received : Outport  Port=2
  CAN_ext : Outport  Port=3
  CAN_id : Outport  Port=4
  CAN_dlc : Outport  Port=5
  CAN_data : Outport  Port=6
  wires:
  In/1 -> mcp2515_read_RX_STATUS/1(In)
  mcp2515_read_RX_STATUS/1(Out) -> Out/1
  checkRxMsgStatus/1(CANRx_Received) -> CAN_Received/1, Relational Operator/1
  mcp2515_read_RX_STATUS/2(RX_STATUS) -> readRxBuffer/1(RX_STATUS), checkRxMsgStatus/1(RX_STATUS)
  readRxBuffer/1(CAN_ext) -> CAN_ext/1
  readRxBuffer/2(CAN_id) -> CAN_id/1
  readRxBuffer/3(CAN_dlc) -> CAN_dlc/1
  readRxBuffer/4(CAN_data) -> CAN_data/1
  CAN_NOMSG/1 -> Relational Operator/2
  Relational Operator/1 -> readRxBuffer/Enable

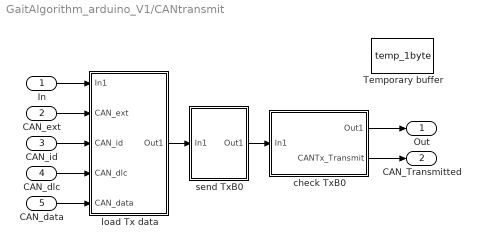
== system GaitAlgorithm_arduino_V1/CANtransmit ==
  In : Inport
  CAN_ext : Inport  Port=2
  CAN_id : Inport  Port=3
  CAN_dlc : Inport  Port=4
  CAN_data : Inport  Port=5
  Temporary buffer : DataStoreMemory  DataStoreName=temp_1byte  ReadBeforeWriteMsg=warning  WriteAfterWriteMsg=warning  WriteAfterReadMsg=warning  ShowAdditionalParam=off  OutDataTypeStr=uint8
  check TxB0 : Subsystem  TreatAsAtomicUnit=on
  load Tx data : Subsystem  TreatAsAtomicUnit=on
  send TxB0 : Subsystem  TreatAsAtomicUnit=on
  Out : Outport
  CAN_Transmitted : Outport  Port=2
  wires:
  In/1 -> load Tx data/1(In1)
  load Tx data/1(Out1) -> send TxB0/1(In1)
  send TxB0/1(Out1) -> check TxB0/1(In1)
  check TxB0/1(Out1) -> Out/1
  check TxB0/2(CANTx_Transmit) -> CAN_Transmitted/1
  CAN_ext/1 -> load Tx data/2(CAN_ext)
  CAN_id/1 -> load Tx data/3(CAN_id)
  CAN_dlc/1 -> load Tx data/4(CAN_dlc)
  CAN_data/1 -> load Tx data/5(CAN_data)

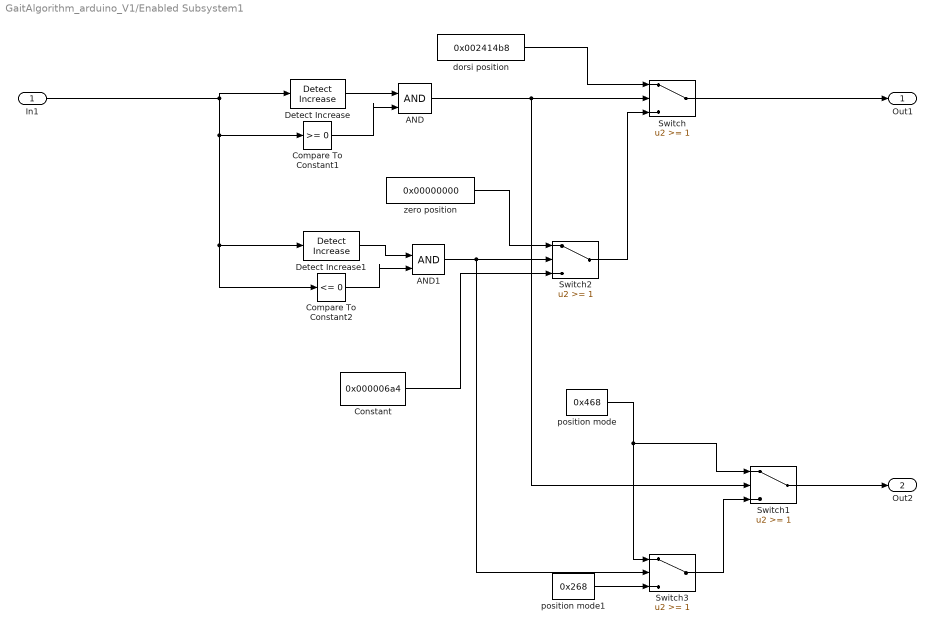
== system GaitAlgorithm_arduino_V1/Enabled Subsystem1 ==
  In1 : Inport
  AND : Logic  IconShape=distinctive  AllPortsSameDT=off  OutDataTypeStr=boolean
  AND1 : Logic  IconShape=distinctive  AllPortsSameDT=off  OutDataTypeStr=boolean
  Compare To Constant1 : simulink/Logic and Bit Operations/Compare To Constant  relop=>=  const=0  OutDataTypeStr=boolean
  Compare To Constant2 : simulink/Logic and Bit Operations/Compare To Constant  relop=<=  const=0  OutDataTypeStr=boolean
  Constant : Constant  Value=0x000006a4
  Detect Increase : simulink/Logic and Bit Operations/Detect Increase  vinit=0.0  OutDataTypeStr=boolean
  Detect Increase1 : simulink/Logic and Bit Operations/Detect Increase  vinit=0.0  OutDataTypeStr=boolean
  Switch{,1..3} (4 alike) : Switch  Threshold=1  OutDataTypeStr=uint32  SaturateOnIntegerOverflow=off  InputSameDT=off
  dorsi position : Constant  Value=0x002414b8
  position mode : Constant  Value=0x468
  position mode1 : Constant  Value=0x268
  zero position : Constant  Value=0x00000000
  Out1 : Outport
  Out2 : Outport  Port=2
  wires:
  In1/1 -> Compare To Constant2/1, Detect Increase1/1, Compare To Constant1/1, Detect Increase/1
  Switch/1 -> Out1/1
  Switch1/1 -> Out2/1
  zero position/1 -> Switch2/1
  Constant/1 -> Switch2/3
  Detect Increase/1 -> AND/1
  Compare To Constant1/1 -> AND/2
  AND/1 -> Switch1/2, Switch/2
  dorsi position/1 -> Switch/1
  Detect Increase1/1 -> AND1/1
  Compare To Constant2/1 -> AND1/2
  AND1/1 -> Switch3/2, Switch2/2
  Switch2/1 -> Switch/3
  position mode/1 -> Switch3/1, Switch1/1
  Switch3/1 -> Switch1/3
  position mode1/1 -> Switch3/3

== system GaitAlgorithm_arduino_V1/Enabled Subsystem3 ==
  In2 : Inport
  Switch4 : Switch  Threshold=1  OutDataTypeStr=uint32  SaturateOnIntegerOverflow=off  InputSameDT=off
  Switch6 : Switch  Threshold=1  OutDataTypeStr=uint32  SaturateOnIntegerOverflow=off  InputSameDT=off
  current brake mode : Constant  Value=[0 0 0x06 0xa4]  OutDataTypeStr=uint8
  current mode2 : Constant  Value=0x268
  plantar : Constant  Value=[0x7f 0xec 0xed 0x30]
  position mode3 : Constant  Value=0x468
  Out1 : Outport
  Out2 : Outport  Port=2
  wires:
  Switch6/1 -> Out2/1
  plantar/1 -> Switch4/1
  current brake mode/1 -> Switch4/3
  position mode3/1 -> Switch6/1
  In2/1 -> Switch6/2, Switch4/2
  current mode2/1 -> Switch6/3
  Switch4/1 -> Out1/1

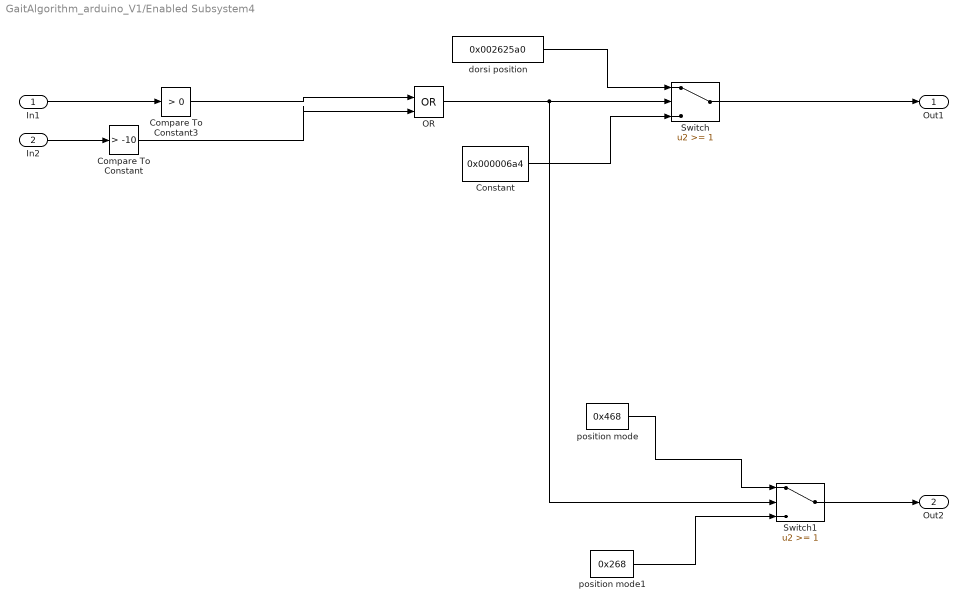
== system GaitAlgorithm_arduino_V1/Enabled Subsystem4 ==
  In1 : Inport
  In2 : Inport  Port=2
  Compare To Constant : simulink/Logic and Bit Operations/Compare To Constant  relop=>  const=-10  OutDataTypeStr=boolean
  Compare To Constant3 : simulink/Logic and Bit Operations/Compare To Constant  relop=>  const=0  OutDataTypeStr=boolean
  Constant : Constant  Value=0x000006a4
  OR : Logic  Operator=OR  IconShape=distinctive  AllPortsSameDT=off  OutDataTypeStr=boolean
  Switch : Switch  Threshold=1  OutDataTypeStr=uint32  SaturateOnIntegerOverflow=off  InputSameDT=off
  Switch1 : Switch  Threshold=1  OutDataTypeStr=uint32  SaturateOnIntegerOverflow=off  InputSameDT=off
  dorsi position : Constant  Value=0x002625a0
  position mode : Constant  Value=0x468
  position mode1 : Constant  Value=0x268
  Out1 : Outport
  Out2 : Outport  Port=2
  wires:
  In1/1 -> Compare To Constant3/1
  Switch/1 -> Out1/1
  Switch1/1 -> Out2/1
  OR/1 -> Switch1/2, Switch/2
  dorsi position/1 -> Switch/1
  Constant/1 -> Switch/3
  position mode/1 -> Switch1/1
  position mode1/1 -> Switch1/3
  In2/1 -> Compare To Constant/1
  Compare To Constant3/1 -> OR/1
  Compare To Constant/1 -> OR/2

== system GaitAlgorithm_arduino_V1/Subsystem ==
  In1 : Inport
  In2 : Inport  Port=2
  In3 : Inport  Port=3
  In5 : Inport  Port=4
  In6 : Inport  Port=5
  Switch1 : Switch  Criteria=u2 > Threshold  Threshold=2  SaturateOnIntegerOverflow=off  InputSameDT=off
  Switch3 : Switch  Criteria=u2 > Threshold  Threshold=1  SaturateOnIntegerOverflow=off  InputSameDT=off
  Switch4 : Switch  Threshold=1  SaturateOnIntegerOverflow=off  InputSameDT=off
  Out1 : Outport
  wires:
  In2/1 -> Switch1/3
  In3/1 -> Switch1/1
  Switch1/1 -> Switch3/1
  Switch3/1 -> Out1/1
  In5/1 -> Switch4/2, Switch1/2, Switch3/2
  Switch4/1 -> Switch3/3
  In1/1 -> Switch4/1
  In6/1 -> Switch4/3

== system GaitAlgorithm_arduino_V1/Subsystem1 ==
  In1 : Inport
  In2 : Inport  Port=2
  In3 : Inport  Port=3
  In5 : Inport  Port=4
  In6 : Inport  Port=5
  Switch1 : Switch  Criteria=u2 > Threshold  Threshold=2  SaturateOnIntegerOverflow=off  InputSameDT=off
  Switch3 : Switch  Criteria=u2 > Threshold  Threshold=1  SaturateOnIntegerOverflow=off  InputSameDT=off
  Switch4 : Switch  Threshold=1  SaturateOnIntegerOverflow=off  InputSameDT=off
  Out1 : Outport
  wires:
  In2/1 -> Switch1/3
  In3/1 -> Switch1/1
  Switch1/1 -> Switch3/1
  Switch3/1 -> Out1/1
  In5/1 -> Switch4/2, Switch1/2, Switch3/2
  Switch4/1 -> Switch3/3
  In1/1 -> Switch4/1
  In6/1 -> Switch4/3

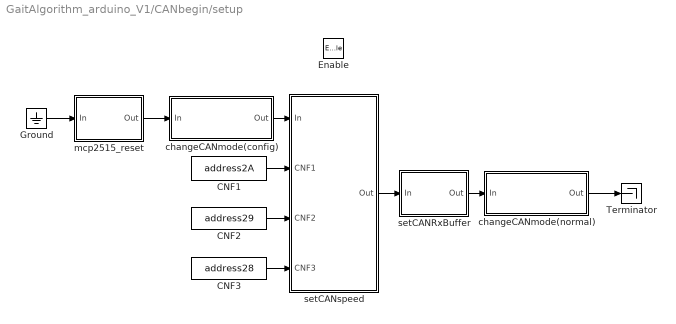
== system GaitAlgorithm_arduino_V1/CANbegin/setup ==
  Enable : EnablePort
  CNF1 : Constant  Value=address2A  OutDataTypeStr=uint8
  CNF2 : Constant  Value=address29  OutDataTypeStr=uint8
  CNF3 : Constant  Value=address28  OutDataTypeStr=uint8
  Ground : Ground
  Terminator : Terminator
  changeCANmode(config) : Subsystem  TreatAsAtomicUnit=on
  changeCANmode(normal) : Subsystem  TreatAsAtomicUnit=on
  mcp2515_reset : Subsystem  TreatAsAtomicUnit=on
  setCANRxBuffer : Subsystem  TreatAsAtomicUnit=on
  setCANspeed : Subsystem  TreatAsAtomicUnit=on
  wires:
  CNF3/1 -> setCANspeed/4(CNF3)
  CNF2/1 -> setCANspeed/3(CNF2)
  CNF1/1 -> setCANspeed/2(CNF1)
  mcp2515_reset/1(Out) -> changeCANmode(config)/1(In)
  changeCANmode(config)/1(Out) -> setCANspeed/1(In)
  setCANspeed/1(Out) -> setCANRxBuffer/1(In)
  setCANRxBuffer/1(Out) -> changeCANmode(normal)/1(In)
  Ground/1 -> mcp2515_reset/1(In)
  changeCANmode(normal)/1(Out) -> Terminator/1

== system GaitAlgorithm_arduino_V1/CANreceive/checkRxMsgStatus ==
  RX_STATUS : Inport
  Bitmask_RxBn : simulink/Logic and Bit Operations/Bitwise Operator  logicop=AND  UseBitMask=on  BitMask=bin2dec('11000000')  BitMaskRealWorld=Stored Integer
  CAN_NOMSG : Constant  Value=-1  OutDataTypeStr=int8
  CAN_OK : Constant  OutDataTypeStr=int8
  Switch : Switch  Criteria=u2 > Threshold  SaturateOnIntegerOverflow=off  InputSameDT=off
  CANRx_Received : Outport
  wires:
  RX_STATUS/1 -> Bitmask_RxBn/1
  CAN_OK/1 -> Switch/1
  CAN_NOMSG/1 -> Switch/3
  Switch/1 -> CANRx_Received/1
  Bitmask_RxBn/1 -> Switch/2

== system GaitAlgorithm_arduino_V1/CANreceive/mcp2515_read_RX_STATUS ==
  In : Inport
  Constant : Constant  Value=0  OutDataTypeStr=uint8
  MCP_RX_STATUS : Constant  Value=hex2dec('B0')  OutDataTypeStr=uint8
  SPI driver : mcp2515lib/CAN application/mcp2515 driver/SPI driver  SystemSampleTime=-1  VariantActivationTime=update diagram  AllowFlexibleInterface=on  Latency=0  AutoFrameSizeCalculation=off
      settings: SourceProductName=CAN device driver for mcp2515
  Selector : Selector  IndexMode=Zero-based  InputPortWidth=2  IndexOptions=Index vector (dialog)  Indices=1  OutputSizes=1
  Vector Concatenate : Concatenate
  Out : Outport
  RX_STATUS : Outport  Port=2
  wires:
  In/1 -> Out/1
  Constant/1 -> Vector Concatenate/2
  SPI driver/1 -> Selector/1
  Selector/1 -> RX_STATUS/1
  MCP_RX_STATUS/1 -> Vector Concatenate/1
  Vector Concatenate/1 -> SPI driver/1

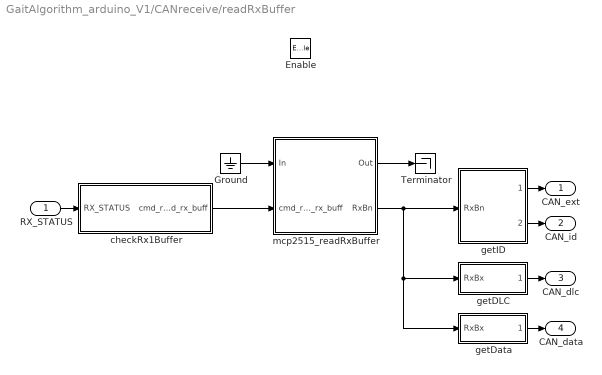
== system GaitAlgorithm_arduino_V1/CANreceive/readRxBuffer ==
  RX_STATUS : Inport
  Enable : EnablePort
  Ground : Ground
  Terminator : Terminator
  checkRx1Buffer : Subsystem  TreatAsAtomicUnit=on
  getDLC : Subsystem  TreatAsAtomicUnit=on
  getData : Subsystem  TreatAsAtomicUnit=on
  getID : Subsystem  TreatAsAtomicUnit=on
      settings: RTWSystemCode=Inline
  mcp2515_readRxBuffer : Subsystem  TreatAsAtomicUnit=on
  CAN_ext : Outport
  CAN_id : Outport  Port=2
  CAN_dlc : Outport  Port=3
  CAN_data : Outport  Port=4
  wires:
  getData/1(CAN_data) -> CAN_data/1
  mcp2515_readRxBuffer/2(RxBn) -> getID/1(RxBn), getData/1(RxBx), getDLC/1(RxBx)
  getID/2(CAN_id) -> CAN_id/1
  getID/1(CAN_ext) -> CAN_ext/1
  getDLC/1(CAN_dlc) -> CAN_dlc/1
  mcp2515_readRxBuffer/1(Out) -> Terminator/1
  Ground/1 -> mcp2515_readRxBuffer/1(In)
  RX_STATUS/1 -> checkRx1Buffer/1(RX_STATUS)
  checkRx1Buffer/1(cmd_read_rx_buff) -> mcp2515_readRxBuffer/2(cmd_read_rx_buff)

== system GaitAlgorithm_arduino_V1/CANtransmit/check TxB0 ==
  In1 : Inport
  Bitmask_TxReq : simulink/Logic and Bit Operations/Bitwise Operator  logicop=AND  UseBitMask=on  BitMask=bin2dec('00001000')  BitMaskRealWorld=Stored Integer
  CAN_FAIL : Constant  Value=2  OutDataTypeStr=int8
  CAN_OK : Constant  OutDataTypeStr=int8
  MCP_TxB0CTRL1 : Constant  Value=hex2dec('30')  OutDataTypeStr=uint8
  Switch : Switch  Criteria=u2 > Threshold  SaturateOnIntegerOverflow=off  InputSameDT=off
  mcp2515_readRegister : Subsystem  TreatAsAtomicUnit=on
  Out1 : Outport
  CANTx_Transmit : Outport  Port=2
  wires:
  CAN_FAIL/1 -> Switch/3
  mcp2515_readRegister/1(Out) -> Out1/1
  mcp2515_readRegister/2(SPI_data) -> Bitmask_TxReq/1
  MCP_TxB0CTRL1/1 -> mcp2515_readRegister/2(address)
  Bitmask_TxReq/1 -> Switch/2
  Switch/1 -> CANTx_Transmit/1
  CAN_OK/1 -> Switch/1
  In1/1 -> mcp2515_readRegister/1(In)

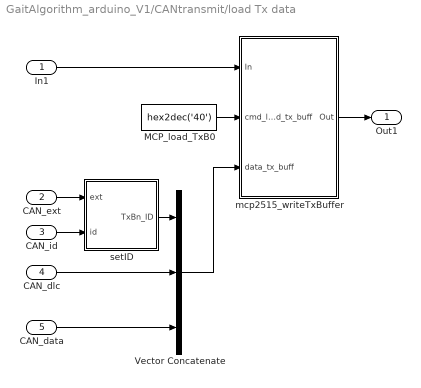
== system GaitAlgorithm_arduino_V1/CANtransmit/load Tx data ==
  In1 : Inport
  CAN_ext : Inport  Port=2
  CAN_id : Inport  Port=3
  CAN_dlc : Inport  Port=4
  CAN_data : Inport  Port=5
  MCP_load_TxB0 : Constant  Value=hex2dec('40')  OutDataTypeStr=uint8
  Vector Concatenate : Concatenate  NumInputs=3
  mcp2515_writeTxBuffer : Subsystem  TreatAsAtomicUnit=on
  setID : Subsystem  TreatAsAtomicUnit=on
      settings: RTWSystemCode=Inline
  Out1 : Outport
  wires:
  CAN_ext/1 -> setID/1(ext)
  CAN_id/1 -> setID/2(id)
  CAN_data/1 -> Vector Concatenate/3
  CAN_dlc/1 -> Vector Concatenate/2
  setID/1(TxBn_ID) -> Vector Concatenate/1
  In1/1 -> mcp2515_writeTxBuffer/1(In)
  mcp2515_writeTxBuffer/1(Out) -> Out1/1
  MCP_load_TxB0/1 -> mcp2515_writeTxBuffer/2(cmd_load_tx_buff)
  Vector Concatenate/1 -> mcp2515_writeTxBuffer/3(data_tx_buff)

== system GaitAlgorithm_arduino_V1/CANtransmit/send TxB0 ==
  In1 : Inport
  MCP_TxB0CTRL : Constant  Value=hex2dec('30')  OutDataTypeStr=uint8
  TxREQ : Constant  Value=8  OutDataTypeStr=uint8
  mcp2515_writeRegister : Subsystem  TreatAsAtomicUnit=on
  Out1 : Outport
  wires:
  MCP_TxB0CTRL/1 -> mcp2515_writeRegister/2(address)
  mcp2515_writeRegister/1(Out) -> Out1/1
  In1/1 -> mcp2515_writeRegister/1(In)
  TxREQ/1 -> mcp2515_writeRegister/3(value)

== system GaitAlgorithm_arduino_V1/CANbegin/setup/changeCANmode(config) ==
  In : Inport
  MCP_CANCTRL : Constant  Value=hex2dec('0F')  OutDataTypeStr=uint8
  MODE_CONFIG : Constant  Value=hex2dec('80')  OutDataTypeStr=uint8
  MODE_MASK : Constant  Value=hex2dec('E0')  OutDataTypeStr=uint8
  mcp2515_modifyRegister : Subsystem  TreatAsAtomicUnit=on
  Out : Outport
  wires:
  MODE_CONFIG/1 -> mcp2515_modifyRegister/4(data)
  MODE_MASK/1 -> mcp2515_modifyRegister/3(mask)
  MCP_CANCTRL/1 -> mcp2515_modifyRegister/2(address)
  In/1 -> mcp2515_modifyRegister/1(In)
  mcp2515_modifyRegister/1(Out) -> Out/1

== system GaitAlgorithm_arduino_V1/CANbegin/setup/changeCANmode(normal) ==
  In : Inport
  MCP_CANCTRL : Constant  Value=hex2dec('0F')  OutDataTypeStr=uint8
  MODE_MASK : Constant  Value=hex2dec('E0')  OutDataTypeStr=uint8
  MODE_NORMAL : Constant  Value=0  OutDataTypeStr=uint8
  mcp2515_modifyRegister : Subsystem  TreatAsAtomicUnit=on
  Out : Outport
  wires:
  MODE_MASK/1 -> mcp2515_modifyRegister/3(mask)
  MODE_NORMAL/1 -> mcp2515_modifyRegister/4(data)
  MCP_CANCTRL/1 -> mcp2515_modifyRegister/2(address)
  In/1 -> mcp2515_modifyRegister/1(In)
  mcp2515_modifyRegister/1(Out) -> Out/1

== system GaitAlgorithm_arduino_V1/CANbegin/setup/mcp2515_reset ==
  In : Inport
  MCP_RESET : Constant  Value=hex2dec('C0')  OutDataTypeStr=uint8
  SPI driver : mcp2515lib/CAN application/mcp2515 driver/SPI driver  SystemSampleTime=-1  VariantActivationTime=update diagram  AllowFlexibleInterface=on  Latency=0  AutoFrameSizeCalculation=off
      settings: SourceProductName=CAN device driver for mcp2515
  Temporary buffer : DataStoreWrite  DataStoreName=temp_1byte  IndexOptions=Index vector (dialog)  Indices=1  OutputSizes=1
  Out : Outport
  wires:
  MCP_RESET/1 -> SPI driver/1
  In/1 -> Out/1
  SPI driver/1 -> Temporary buffer/1

== system GaitAlgorithm_arduino_V1/CANbegin/setup/setCANRxBuffer ==
  note: RXB0
  note: RXB1
  note: no filter, no mask
  In : Inport
  MCP_RXB0CTRL : Constant  Value=hex2dec('60')  OutDataTypeStr=uint8
  MCP_RXB1CTRL : Constant  Value=hex2dec('70')  OutDataTypeStr=uint8
  MCP_RXB_RX_MASK : Constant  Value=hex2dec('60')  OutDataTypeStr=uint8
  mcp2515_writeRegister : Subsystem  TreatAsAtomicUnit=on
  mcp2515_writeRegister1 : Subsystem  TreatAsAtomicUnit=on
  Out : Outport
  wires:
  MCP_RXB0CTRL/1 -> mcp2515_writeRegister/2(address)
  MCP_RXB1CTRL/1 -> mcp2515_writeRegister1/2(address)
  MCP_RXB_RX_MASK/1 -> mcp2515_writeRegister1/3(value), mcp2515_writeRegister/3(value)
  In/1 -> mcp2515_writeRegister/1(In)
  mcp2515_writeRegister1/1(Out) -> Out/1
  mcp2515_writeRegister/1(Out) -> mcp2515_writeRegister1/1(In)

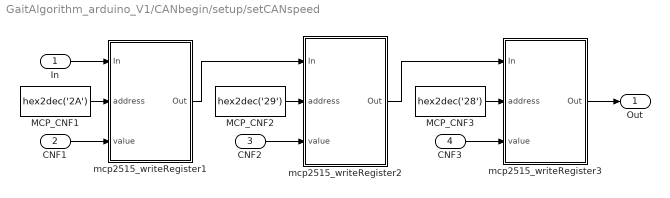
== system GaitAlgorithm_arduino_V1/CANbegin/setup/setCANspeed ==
  In : Inport
  CNF1 : Inport  Port=2
  CNF2 : Inport  Port=3
  CNF3 : Inport  Port=4
  MCP_CNF1 : Constant  Value=hex2dec('2A')  OutDataTypeStr=uint8
  MCP_CNF2 : Constant  Value=hex2dec('29')  OutDataTypeStr=uint8
  MCP_CNF3 : Constant  Value=hex2dec('28')  OutDataTypeStr=uint8
  mcp2515_writeRegister1 : Subsystem  TreatAsAtomicUnit=on
  mcp2515_writeRegister2 : Subsystem  TreatAsAtomicUnit=on
  mcp2515_writeRegister3 : Subsystem  TreatAsAtomicUnit=on
  Out : Outport
  wires:
  MCP_CNF2/1 -> mcp2515_writeRegister2/2(address)
  MCP_CNF3/1 -> mcp2515_writeRegister3/2(address)
  CNF3/1 -> mcp2515_writeRegister3/3(value)
  CNF1/1 -> mcp2515_writeRegister1/3(value)
  MCP_CNF1/1 -> mcp2515_writeRegister1/2(address)
  CNF2/1 -> mcp2515_writeRegister2/3(value)
  In/1 -> mcp2515_writeRegister1/1(In)
  mcp2515_writeRegister1/1(Out) -> mcp2515_writeRegister2/1(In)
  mcp2515_writeRegister2/1(Out) -> mcp2515_writeRegister3/1(In)
  mcp2515_writeRegister3/1(Out) -> Out/1

== system GaitAlgorithm_arduino_V1/CANreceive/readRxBuffer/checkRx1Buffer ==
  RX_STATUS : Inport
  Bitmask_RxB1_Status : simulink/Logic and Bit Operations/Bitwise Operator  logicop=AND  UseBitMask=on  BitMask=bin2dec('10000000')  BitMaskRealWorld=Stored Integer
  MCP_READ_RxB0 : Constant  Value=hex2dec('90')  OutDataTypeStr=uint8
  MCP_READ_RxB1 : Constant  Value=hex2dec('94')  OutDataTypeStr=uint8
  Switch : Switch  Criteria=u2 > Threshold  SaturateOnIntegerOverflow=off  InputSameDT=off
  cmd_read_rx_buff : Outport
  wires:
  Switch/1 -> cmd_read_rx_buff/1
  MCP_READ_RxB1/1 -> Switch/1
  MCP_READ_RxB0/1 -> Switch/3
  Bitmask_RxB1_Status/1 -> Switch/2
  RX_STATUS/1 -> Bitmask_RxB1_Status/1
